simulink model "Sim_Modell_hydraulisches_System"  (R2020b)
settings: Solver=ode15s  StartTime=0.0  StopTime=10  RelTol=1e-6  AbsTol=1e-5  EnableMultiTasking=on
undefined symbols (not defined in the file or in its folder): parImp, parRegA, parRegoA, parSys
libraries: simulink x5, cstblocks x2
settings Model: Creator=wke  LastModifiedBy=Simon
settings SolverCC: AutoScaleAbsTol=off
settings DataIOCC: LimitDataPoints=on  SaveFormat=Array  SignalLoggingSaveFormat=ModelDataLogs  ReturnWorkspaceOutputs=off
settings OptimizationCC: ExpressionDepthLimit=2147483647  InitFltsAndDblsToZero=on  LifeSpan=inf
settings DebuggingCC: UnderspecifiedInitializationDetection=Classic  MergeDetectMultiDrivingBlocksExec=none  SolverPrmCheckMsg=warning  FcnCallInpInsideContextMsg=warning  StateNameClashWarn=warning  SFUnexpectedBacktrackingDiag=warning  SFNoUnconditionalDefaultTransitionDiag=warning  SFExecutionAtInitializationDiag=none  ArithmeticOperatorsInVariantConditions=warning
settings HardwareCC: ProdBitPerPointer=32  ProdBitPerSizeT=32  ProdBitPerPtrDiffT=32  ProdLargestAtomicFloat=None  ProdIntDivRoundTo=Undefined  ProdEndianess=Unspecified  ProdWordSize=32  ProdHWDeviceType=32-bit Generic
settings ModelReferenceCC: PropagateSignalLabelsOutOfModel=off
settings SFSimCC: SimUseLocalCustomCode=off  SimParseCustomCode=off  CustomCodeUndefinedFunction=UseInterfaceOnly
settings RTWCC: RTWUseLocalCustomCode=off
settings CodeAppCC: StateflowObjectComments=on
settings GRTTargetCC: TargetLangStandard=C89/C90 (ANSI)  CombineOutputUpdateFcns=off  GRTInterface=on
settings ConfigComp: CovMetricSettings=dw  CovSaveCumulativeToWorkspaceVar=on  CovSaveSingleToWorkspaceVar=on  CovExternalEMLEnable=off

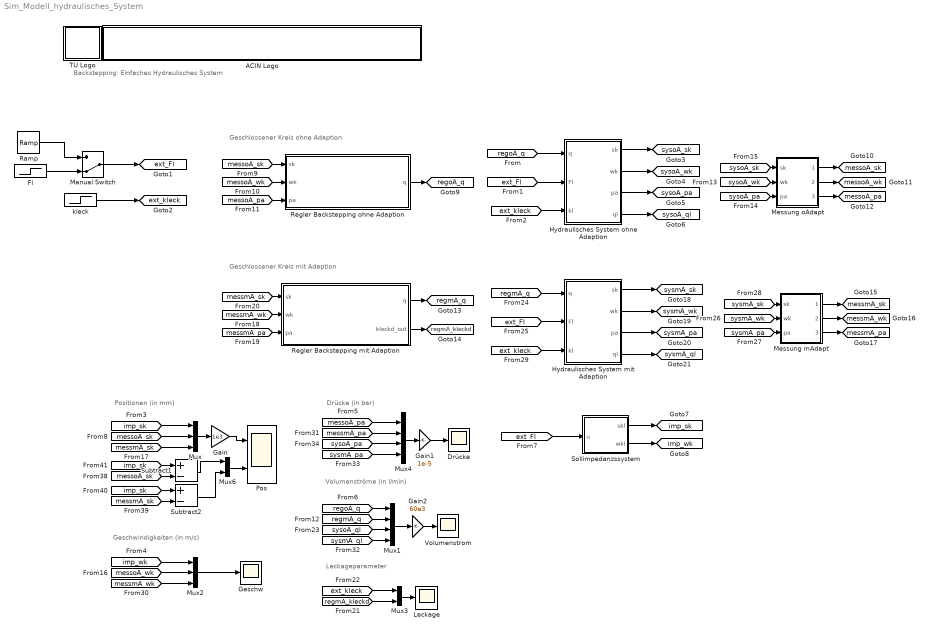
== system Sim_Modell_hydraulisches_System ==
  note: Positionen (in mm)
  note: Geschwindigkeiten (in m/s)
  note: Drücke (in bar)
  note: Leckageparameter
  note: Volumenströme (in l/min)
  note: Geschlossener Kreis ohne Adaption
  note: Geschlossener Kreis mit Adaption
  note: Backstepping: Einfaches Hydraulisches System
  ACIN Logo : Subsystem
      mask init:
      | s = get_param(gcb,'UserData');
      mask Display:
      | image(s.logo,[0 0 439 45]);
      | %axis image
  Drücke : Scope
  Fl : Step  Time=5  After=1e3*1  SampleTime=0
  Gain : Gain  Gain=1e3
  Gain1 : Gain  Gain=1e-5
  Gain2 : Gain  Gain=60e3
  Geschw : Scope
  "Hydraulisches System mit Adaption " : Subsystem
  Hydraulisches System ohne Adaption : Subsystem
  Leckage : Scope
  Manual Switch : ManualSwitch  CurrentSetting=0
  Messung mAdapt : Subsystem  mask{rauschenein_par=on, rauschampl_sk=5e-4, rauschampl_pa=5e4}
      mask prompts: rauschenein_par "Rauschen ein"; rauschampl_sk "Rauschamplitude Position sk"; rauschampl_pa "Rauschamplitude Druck pa"
  Messung oAdapt : Subsystem  mask{rauschenein_par=on, rauschampl_sk=5e-4, rauschampl_pa=5e4}
      mask prompts: rauschenein_par "Rauschen ein"; rauschampl_sk "Rauschamplitude Position sk"; rauschampl_pa "Rauschamplitude Druck pa"
  Mux : Mux  Inputs=3
  Mux1 : Mux
  Mux2 : Mux  Inputs=3
  Mux3 : Mux  Inputs=2
  Mux4 : Mux
  Mux6 : Mux  Inputs=2
  Pos : Scope  NumInputPorts=2
  Ramp : simulink/Sources/Ramp  slope=200  start=0  InitialOutput=0
  Regler Backstepping mit Adaption : MATLAB Function
  Regler Backstepping ohne Adaption : MATLAB Function  TreatAsAtomicUnit=on
  Sollimpedanzssystem : Subsystem
  Subtract1 : Sum  Inputs=+-
  Subtract2 : Sum  Inputs=+-
  TU Logo : Subsystem
      mask init:
      | s = get_param(gcb,'UserData');
      mask Display: image(s.logo,[0 0 45 45]);
  Volumenstrom : Scope
  kleck : Step  Before=parSys.klecknom*1  After=parSys.klecknom*2  SampleTime=0
  tag scope: ext_Fl=global, ext_kleck=global, imp_sk=global, imp_wk=global, messmA_pa=global, messmA_sk=global, messmA_wk=global, messoA_pa=global, messoA_sk=global, messoA_wk=global, regmA_kleckd=global, regmA_q=global, regoA_q=global, sysmA_pa=global, sysmA_ql=global, sysmA_sk=global, sysmA_wk=global, sysoA_pa=global, sysoA_ql=global, sysoA_sk=global, sysoA_wk=global
  wires:
  [regoA_q] -> Hydraulisches System ohne Adaption/1(q)
  kleck/1 -> [ext_kleck]
  [ext_Fl] -> Hydraulisches System ohne Adaption/2(Fl)
  [ext_kleck] -> Hydraulisches System ohne Adaption/3(kl)
  Hydraulisches System ohne Adaption/1(sk) -> [sysoA_sk]
  Hydraulisches System ohne Adaption/2(wk) -> [sysoA_wk]
  Hydraulisches System ohne Adaption/3(pa) -> [sysoA_pa]
  Gain/1 -> Pos/1
  Gain1/1 -> Drücke/1
  Gain2/1 -> Volumenstrom/1
  Mux/1 -> Gain/1
  [imp_sk] -> Mux/1
  Regler Backstepping ohne Adaption/1(q) -> [regoA_q]
  [messoA_wk] -> Regler Backstepping ohne Adaption/2(wk)
  [messoA_sk] -> Regler Backstepping ohne Adaption/1(sk)
  [messoA_pa] -> Regler Backstepping ohne Adaption/3(pa)
  [regoA_q] -> Mux1/1
  Mux1/1 -> Gain2/1
  [regmA_q] -> Mux1/2
  [sysoA_sk] -> Messung oAdapt/1(sk)
  [sysoA_wk] -> Messung oAdapt/2(wk)
  [sysoA_pa] -> Messung oAdapt/3(pa)
  Messung oAdapt/3(pamess) -> [messoA_pa]
  Messung oAdapt/2(wkmess) -> [messoA_wk]
  Messung oAdapt/1(skmess) -> [messoA_sk]
  [imp_wk] -> Mux2/1
  Mux2/1 -> Geschw/1
  [messoA_wk] -> Mux2/2
  [messmA_sk] -> Mux/3
  [messmA_wk] -> Regler Backstepping mit Adaption/2(wk)
  [messmA_sk] -> Regler Backstepping mit Adaption/1(sk)
  [messmA_pa] -> Regler Backstepping mit Adaption/3(pa)
  Regler Backstepping mit Adaption/2(kleckd_out) -> [regmA_kleckd]
  Regler Backstepping mit Adaption/1(q) -> [regmA_q]
  [ext_kleck] -> Mux3/1
  Mux3/1 -> Leckage/1
  [regmA_kleckd] -> Mux3/2
  [sysoA_ql] -> Mux1/3
  [regmA_q] -> "Hydraulisches System mit Adaption "/1(q)
  [ext_Fl] -> "Hydraulisches System mit Adaption "/2(Fl)
  [ext_kleck] -> "Hydraulisches System mit Adaption "/3(kl)
  "Hydraulisches System mit Adaption "/1(sk) -> [sysmA_sk]
  "Hydraulisches System mit Adaption "/2(wk) -> [sysmA_wk]
  "Hydraulisches System mit Adaption "/4(ql) -> [sysmA_ql]
  [sysmA_sk] -> Messung mAdapt/1(sk)
  [sysmA_wk] -> Messung mAdapt/2(wk)
  [sysmA_pa] -> Messung mAdapt/3(pa)
  Messung mAdapt/3(pamess) -> [messmA_pa]
  Messung mAdapt/2(wkmess) -> [messmA_wk]
  Messung mAdapt/1(skmess) -> [messmA_sk]
  [messmA_wk] -> Mux2/3
  [messoA_pa] -> Mux4/1
  [messmA_pa] -> Mux4/2
  Mux4/1 -> Gain1/1
  [sysmA_ql] -> Mux1/4
  [sysoA_pa] -> Mux4/3
  [sysmA_pa] -> Mux4/4
  Hydraulisches System ohne Adaption/4(ql) -> [sysoA_ql]
  "Hydraulisches System mit Adaption "/3(pa) -> [sysmA_pa]
  [imp_sk] -> Subtract1/1
  [messoA_sk] -> Subtract1/2
  [imp_sk] -> Subtract2/1
  [messmA_sk] -> Subtract2/2
  Subtract2/1 -> Mux6/2
  Subtract1/1 -> Mux6/1
  Mux6/1 -> Pos/2
  [ext_Fl] -> Sollimpedanzssystem/1(u)
  Sollimpedanzssystem/1(skl) -> [imp_sk]
  Sollimpedanzssystem/2(wkl) -> [imp_wk]
  [messoA_sk] -> Mux/2
  Manual Switch/1 -> [ext_Fl]
  Fl/1 -> Manual Switch/2
  Ramp/1 -> Manual Switch/1

== system Sim_Modell_hydraulisches_System/ACIN Logo ==

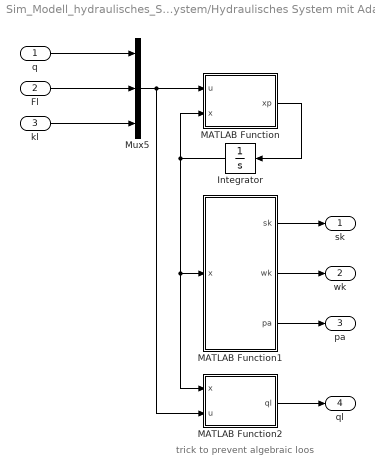
== system Sim_Modell_hydraulisches_System/Hydraulisches System mit Adaption  ==
  note: trick to prevent algebraic loos
  q : Inport
  Fl : Inport  Port=2
  kl : Inport  Port=3
  Integrator : Integrator  InitialCondition=[parSys.sk0; parSys.wk0; parSys.pa0]
  MATLAB Function : MATLAB Function  TreatAsAtomicUnit=on
  MATLAB Function1 : MATLAB Function  TreatAsAtomicUnit=on
  MATLAB Function2 : MATLAB Function  TreatAsAtomicUnit=on
  Mux5 : Mux  Inputs=3
  sk : Outport
  wk : Outport  Port=2
  pa : Outport  Port=3
  ql : Outport  Port=4
  wires:
  MATLAB Function1/2(wk) -> wk/1
  MATLAB Function1/3(pa) -> pa/1
  Mux5/1 -> MATLAB Function2/2(u), MATLAB Function/1(u)
  MATLAB Function/1(xp) -> Integrator/1
  MATLAB Function1/1(sk) -> sk/1
  Fl/1 -> Mux5/2
  kl/1 -> Mux5/3
  Integrator/1 -> MATLAB Function/2(x), MATLAB Function2/1(x), MATLAB Function1/1(x)
  q/1 -> Mux5/1
  MATLAB Function2/1(ql) -> ql/1

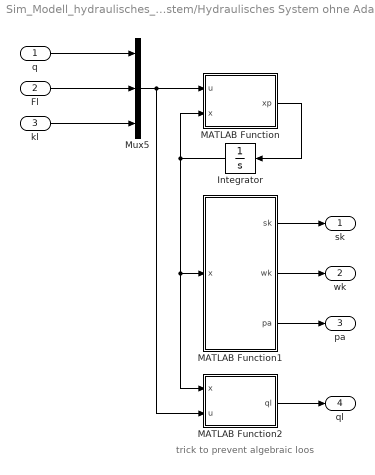
== system Sim_Modell_hydraulisches_System/Hydraulisches System ohne Adaption ==
  note: trick to prevent algebraic loos
  q : Inport
  Fl : Inport  Port=2
  kl : Inport  Port=3
  Integrator : Integrator  InitialCondition=[parSys.sk0; parSys.wk0; parSys.pa0]
  MATLAB Function : MATLAB Function  TreatAsAtomicUnit=on
  MATLAB Function1 : MATLAB Function  TreatAsAtomicUnit=on
  MATLAB Function2 : MATLAB Function  TreatAsAtomicUnit=on
  Mux5 : Mux  Inputs=3
  sk : Outport
  wk : Outport  Port=2
  pa : Outport  Port=3
  ql : Outport  Port=4
  wires:
  MATLAB Function1/2(wk) -> wk/1
  MATLAB Function1/3(pa) -> pa/1
  Mux5/1 -> MATLAB Function2/2(u), MATLAB Function/1(u)
  MATLAB Function/1(xp) -> Integrator/1
  MATLAB Function1/1(sk) -> sk/1
  Fl/1 -> Mux5/2
  kl/1 -> Mux5/3
  Integrator/1 -> MATLAB Function/2(x), MATLAB Function2/1(x), MATLAB Function1/1(x)
  q/1 -> Mux5/1
  MATLAB Function2/1(ql) -> ql/1

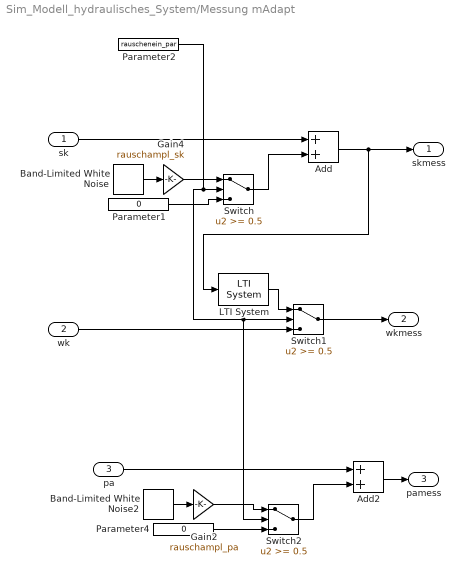
== system Sim_Modell_hydraulisches_System/Messung mAdapt ==
  sk : Inport
  wk : Inport  Port=2
  pa : Inport  Port=3
  Add : Sum
  Add2 : Sum
  Band-Limited White Noise : simulink/Sources/Band-Limited White Noise  Cov=[0.0001]  Ts=0.001  seed=[23341]
  Band-Limited White Noise2 : simulink/Sources/Band-Limited White Noise  Cov=[0.0001]  Ts=0.001  seed=[23341]
  Gain2 : Gain  Gain=rauschampl_pa
  Gain4 : Gain  Gain=rauschampl_sk
  LTI System : cstblocks/LTI System  sys=parMess.Gdiffsk  IC=[]
  Parameter1 : Constant  Value=0  VectorParams1D=off
  Parameter2 : Constant  Value=rauschenein_par  VectorParams1D=off
  Parameter4 : Constant  Value=0  VectorParams1D=off
  Switch : Switch  Threshold=0.5
  Switch1 : Switch  Threshold=0.5
  Switch2 : Switch  Threshold=0.5
  skmess : Outport
  wkmess : Outport  Port=2
  pamess : Outport  Port=3
  wires:
  Parameter1/1 -> Switch/3
  Gain4/1 -> Switch/1
  wk/1 -> Switch1/3
  LTI System/1 -> Switch1/1
  Gain2/1 -> Switch2/1
  Parameter4/1 -> Switch2/3
  Switch1/1 -> wkmess/1
  Add2/1 -> pamess/1
  pa/1 -> Add2/1
  Switch2/1 -> Add2/2
  Band-Limited White Noise2/1 -> Gain2/1
  Add/1 -> LTI System/1, skmess/1
  sk/1 -> Add/1
  Parameter2/1 -> Switch2/2, Switch1/2, Switch/2
  Switch/1 -> Add/2
  Band-Limited White Noise/1 -> Gain4/1

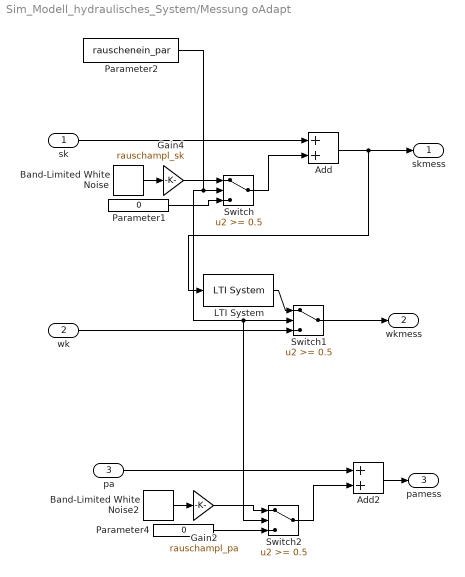
== system Sim_Modell_hydraulisches_System/Messung oAdapt ==
  sk : Inport
  wk : Inport  Port=2
  pa : Inport  Port=3
  Add : Sum
  Add2 : Sum
  Band-Limited White Noise : simulink/Sources/Band-Limited White Noise  Cov=[0.0001]  Ts=0.001  seed=[23341]
  Band-Limited White Noise2 : simulink/Sources/Band-Limited White Noise  Cov=[0.0001]  Ts=0.001  seed=[23341]
  Gain2 : Gain  Gain=rauschampl_pa
  Gain4 : Gain  Gain=rauschampl_sk
  LTI System : cstblocks/LTI System  sys=parMess.Gdiffsk  IC=[]
  Parameter1 : Constant  Value=0  VectorParams1D=off
  Parameter2 : Constant  Value=rauschenein_par  VectorParams1D=off
  Parameter4 : Constant  Value=0  VectorParams1D=off
  Switch : Switch  Threshold=0.5
  Switch1 : Switch  Threshold=0.5
  Switch2 : Switch  Threshold=0.5
  skmess : Outport
  wkmess : Outport  Port=2
  pamess : Outport  Port=3
  wires:
  Band-Limited White Noise/1 -> Gain4/1
  Switch/1 -> Add/2
  Parameter2/1 -> Switch/2, Switch1/2, Switch2/2
  sk/1 -> Add/1
  Add/1 -> skmess/1, LTI System/1
  Band-Limited White Noise2/1 -> Gain2/1
  Switch2/1 -> Add2/2
  pa/1 -> Add2/1
  Add2/1 -> pamess/1
  Switch1/1 -> wkmess/1
  Parameter4/1 -> Switch2/3
  Gain2/1 -> Switch2/1
  LTI System/1 -> Switch1/1
  wk/1 -> Switch1/3
  Gain4/1 -> Switch/1
  Parameter1/1 -> Switch/3

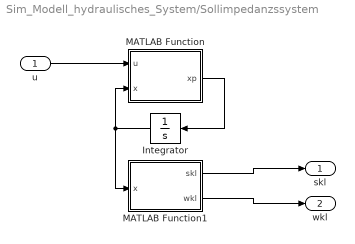
== system Sim_Modell_hydraulisches_System/Sollimpedanzssystem ==
  u : Inport
  Integrator : Integrator  InitialCondition=[parSys.sk0; parSys.wk0]
  MATLAB Function : MATLAB Function  TreatAsAtomicUnit=on
  MATLAB Function1 : MATLAB Function  TreatAsAtomicUnit=on
  skl : Outport
  wkl : Outport  Port=2
  wires:
  MATLAB Function1/2(wkl) -> wkl/1
  MATLAB Function/1(xp) -> Integrator/1
  u/1 -> MATLAB Function/1(u)
  MATLAB Function1/1(skl) -> skl/1
  Integrator/1 -> MATLAB Function1/1(x), MATLAB Function/2(x)

== system Sim_Modell_hydraulisches_System/TU Logo ==

== matlab function Sim_Modell_hydraulisches_System/Sollimpedanzssystem/MATLAB Function1 ==
  data: x input; skl output; wkl output
function [skl, wkl] = h(x)

skl = x(1);
wkl = x(2);

== matlab function Sim_Modell_hydraulisches_System/Regler Backstepping mit Adaption ==
  settings: updateMethod=DISCRETE  sampleTime=parRegA.Ts
  data sk settings: updateMethod=SF_CONTINUOUS_TIME_DATA
  data wk settings: updateMethod=SF_CONTINUOUS_TIME_DATA
  data pa settings: updateMethod=SF_CONTINUOUS_TIME_DATA
  data parSys settings: updateMethod=SF_CONTINUOUS_TIME_DATA
  data q settings: updateMethod=SF_CONTINUOUS_TIME_DATA
  data: sk input; wk input; pa input; parSys parameter; q output; kleckd_out output; parImp parameter; parRegA parameter
function [q,kleckd_out]  = Backstepping_mit_Adapt(sk,wk,pa,parSys,parImp, parRegA)
% Funktion zur Implementierung eines Backsteppingreglers mit
% Adaption für einfaches hydraulisches System


% Initialisierung des diskreten Integrator Zustandes
persistent kleckd
if isempty(kleckd) kleckd = parSys.klecknom; end

% Zuweisung der Parameter

m = parSys.m;
dk = parSys.dk;
beta = parSys.beta;
Aa = parSys.Aa;
Ab = parSys.Ab;
V0a = parSys.V0a;
pb = parSys.pb;


c1I = parImp.c1I;
c3I = parImp.c3I;
c0I= parImp.c0I;
skImax = parImp.skImax;
d1I = parImp.d1I;
numFeder = parImp.numFeder;

k0=parRegA.k0;
k1= parRegA.k1;
gamma = parRegA.gamma;

%Berechnung von Fp aus pa und pb
Fp=pa*Aa-pb*Ab;

%Berechnung der Einträge des Systems
f1=[wk;-dk/m*wk];
g1=[0;1/m];
f2dach=[beta*Aa/(V0a+Aa*sk)*(-Aa*wk-kleckd/Aa*(Fp-pb*(Aa-Ab)))];
g2=[beta*Aa/(V0a+Aa*sk)];
x1=[sk;wk];
x2=[Fp];

%Bestimmung der Federkraft und der Ableitung der Federkraft
if numFeder<1.5
    FcI=c1I*sk;      %lineare Feder
    dFcIdsk=c1I;
elseif numFeder<2.5
    FcI=c1I*sk+c3I*sk^3;
    dFcIdsk=c1I+3*c3I*sk^2;
else
    FcI=c0I*2*skImax/pi*tan(pi*sk/2/skImax);
    dFcIdsk=c0I*(1+(tan(pi*sk/2/skImax))^2);
end;

%Berechnung von alpha1 und dalpha1/dx1
alpha1=-FcI-(d1I-dk)*wk;
dalpha1dx1=[-dFcIdsk,-(d1I-dk)];

%Berechnung von dV1dx1
dV1dx1=[FcI,m*wk];

%Berechnung des Stellgesetzes
q=1/g2*(-f2dach+dalpha1dx1*(f1+g1*x2)-dV1dx1*g1/gamma-k1*(x2-alpha1));

%Berechnung des Parameterschätzers
kleckd_out = kleckd; % Ausgabe des aktuellen Zustandes

chi=beta/(V0a+Aa*sk)*(Fp-pb*(Aa-Ab));
dkleckddt=-k0*(x2-alpha1)*chi;
% Zeitdiskreter Intergratorschritt nach Euler-Vorwärts
kleckd = kleckd + parRegA.Ts*dkleckddt;

== matlab function Sim_Modell_hydraulisches_System/Regler Backstepping ohne Adaption ==
  data sk settings: updateMethod=SF_CONTINUOUS_TIME_DATA
  data wk settings: updateMethod=SF_CONTINUOUS_TIME_DATA
  data pa settings: updateMethod=SF_CONTINUOUS_TIME_DATA
  data parSys settings: updateMethod=SF_CONTINUOUS_TIME_DATA
  data q settings: updateMethod=SF_CONTINUOUS_TIME_DATA
  data: sk input; wk input; pa input; parSys parameter; q output; parRegoA parameter; parImp parameter
function q  = Backstepping_ohne_Adapt(sk,wk,pa,parSys, parRegoA, parImp)
% Funktion zur Implementierung eines Backsteppingreglers ohne
% Adaption für einfaches hydraulisches System

% Zuweisung der Parameter

m = parSys.m;
dk = parSys.dk;
beta = parSys.beta;
Aa = parSys.Aa;
Ab = parSys.Ab;
V0a = parSys.V0a;
pb = parSys.pb;
klecknom = parSys.klecknom;

c1I = parImp.c1I;
c3I = parImp.c3I;
c0I= parImp.c0I;
skImax = parImp.skImax;
d1I = parImp.d1I;
numFeder = parImp.numFeder;

k1= parRegoA.k1;
gamma = parRegoA.gamma;

%Berechnung von Fp aus pa und pb
Fp=pa*Aa-pb*Ab;

%Berechnung der Einträge des Systems
f1=[wk;-dk/m*wk];
g1=[0;1/m];
f2=[beta*Aa/(V0a+Aa*sk)*(-Aa*wk-klecknom/Aa*(Fp-pb*(Aa-Ab)))];
g2=[beta*Aa/(V0a+Aa*sk)];
x1=[sk;wk];
x2=[Fp];

%Bestimmung der Federkraft und der Ableitung der Federkraft
if numFeder<1.5
    FcI=c1I*sk;      %lineare Feder
    dFcIdsk=c1I;
elseif numFeder<2.5
    FcI=c1I*sk+c3I*sk^3;
    dFcIdsk=c1I+3*c3I*sk^2;
else
    FcI=c0I*2*skImax/pi*tan(pi*sk/2/skImax);
    dFcIdsk=c0I*(1+(tan(pi*sk/2/skImax))^2);
end;

%Berechnung von alpha1 und dalpha1/dx1
alpha1=-FcI-(d1I-dk)*wk;
dalpha1dx1=[-dFcIdsk,-(d1I-dk)];

%Berechnung von dV1dx1
 dV1dx1=[FcI,m*wk];


%Berechnung des Stellgesetzes
q=1/g2*(-f2+dalpha1dx1*(f1+g1*x2)-dV1dx1*g1/gamma-k1*(x2-alpha1));

== matlab function Sim_Modell_hydraulisches_System/Hydraulisches System mit Adaption /MATLAB Function ==
  data: u input; x input; xp output; parSys parameter
function xp = f(u,x,parSys)

xp = zeros(3,1); % necessary for defining the size


% map parameter
Aa_par   	= parSys.Aa;
Ab_par      = parSys.Ab;
V0a_par     = parSys.V0a;
pb_par      = parSys.pb;
beta_par    = parSys.beta;
dk_par      = parSys.dk;
m_par       = parSys.m;

%  map inputs and states
q  = u(1);
Fl = u(2);
kl = u(3);

sk = x(1);
wk = x(2);
pa = x(3);

%     /* leakage flow */
ql = kl*(pa-pb_par);

%   /* derivatives */
xp = [wk;
      1/m_par*(pa*Aa_par-pb_par*Ab_par-dk_par*wk-Fl);
      beta_par/(V0a_par+Aa_par*sk)*(-Aa_par*wk-ql+q);];

== matlab function Sim_Modell_hydraulisches_System/Hydraulisches System mit Adaption /MATLAB Function1 ==
  data: x input; sk output; parSys parameter; wk output; pa output
function [sk,wk,pa] = h1(x,parSys)

% necesarry for simulink automatic dimension detection
sk = 0;
wk = 0;
pa = 0;

%q  = u(1);
%Fl = u(2);
%kl = u(3);

% define the outputs
sk = x(1);
wk = x(2);
pa = x(3);


end

== matlab function Sim_Modell_hydraulisches_System/Hydraulisches System ohne Adaption/MATLAB Function ==
  data: u input; x input; xp output; parSys parameter
function xp = f(u,x,parSys)

xp = zeros(3,1); % necessary for defining the size


% map parameter
Aa_par   	= parSys.Aa;
Ab_par      = parSys.Ab;
V0a_par     = parSys.V0a;
pb_par      = parSys.pb;
beta_par    = parSys.beta;
dk_par      = parSys.dk;
m_par       = parSys.m;

%  map inputs and states
q  = u(1);
Fl = u(2);
kl = u(3);

sk = x(1);
wk = x(2);
pa = x(3);

%     /* leakage flow */
ql = kl*(pa-pb_par);

%   /* derivatives */
xp = [wk;
      1/m_par*(pa*Aa_par-pb_par*Ab_par-dk_par*wk-Fl);
      beta_par/(V0a_par+Aa_par*sk)*(-Aa_par*wk-ql+q);];

== matlab function Sim_Modell_hydraulisches_System/Hydraulisches System ohne Adaption/MATLAB Function1 ==
  data: x input; sk output; parSys parameter; wk output; pa output
function [sk,wk,pa] = h1(x,parSys)

% necesarry for simulink automatic dimension detection
sk = 0;
wk = 0;
pa = 0;

%q  = u(1);
%Fl = u(2);
%kl = u(3);

% define the outputs
sk = x(1);
wk = x(2);
pa = x(3);


end

== matlab function Sim_Modell_hydraulisches_System/Hydraulisches System mit Adaption /MATLAB Function2 ==
  data: x input; u input; ql output; parSys parameter
function ql = h2(x,u,parSys)

% map parameters
pb_par      = parSys.pb;

% map inputs
kl = u(3);

% map states
pa = x(3);

% calculate outputs
ql = kl*(pa-pb_par);

== matlab function Sim_Modell_hydraulisches_System/Hydraulisches System ohne Adaption/MATLAB Function2 ==
  data: x input; u input; ql output; parSys parameter
function ql = h2(x,u,parSys)

% map parameters
pb_par      = parSys.pb;

% map inputs
kl = u(3);

% map states
pa = x(3);

% calculate outputs
ql = kl*(pa-pb_par);

== matlab function Sim_Modell_hydraulisches_System/Sollimpedanzssystem/MATLAB Function ==
  data: u input; xp output; x input; parImp parameter; parSys parameter
function xp = f(u,x, parImp, parSys)

xp = zeros(2,1);

% map parameters
m_par   	= parSys.m;
c1I_par     = parImp.c1I;
c3I_par     = parImp.c3I;
c0I_par     = parImp.c0I;
skImax_par  = parImp.skImax;
numFeder_par= parImp.numFeder;
d1I_par     = parImp.d1I;


% map inputs and states
skI = x(1);
wkI = x(2);
Fl = u;


%  calculate spring force
if numFeder_par<0.5 
    error('unknown spring form');
elseif  numFeder_par<1.5 
    Fc = c1I_par*skI;    % /* linear spring*/
elseif numFeder_par<2.5    
    Fc = c1I_par*skI+c3I_par*skI^3;   % /* cubic spring */
elseif numFeder_par<3.5
    Fc = c0I_par*2.0*skImax_par/pi*tan(pi*skI/2.0/skImax_par); % /* tan spring*/
else
    error('unknown spring form');
end

% derivatives
xp(1) = wkI;
xp(2) = 1/m_par*(-Fc-d1I_par*wkI-Fl);
